simulink model "ServoModel_v5"  (R2021b)
settings: Solver=FixedStepAuto  StartTime=0.0  StopTime=Inf  RelTol=1e-3  EnableMultiTasking=on
libraries: simulink x1, arduinolib x1
settings Model: ExtModeTrigDuration=2  Creator=diego  LastModifiedBy=diego
settings OptimizationCC: EnhancedBackFolding=on  PassReuseOutputArgsAs=Individual arguments  ZeroExternalMemoryAtStartup=off  ZeroInternalMemoryAtStartup=off  MaxStackSize=64  OptimizeBlockOrder=speed  DifferentSizesBufferReuse=on  EfficientTunableParamExpr=on
settings DebuggingCC: ParameterTunabilityLossMsg=error
settings HardwareCC: ProdBitPerInt=16  ProdBitPerPointer=16  ProdBitPerSizeT=16  ProdBitPerPtrDiffT=16  ProdLargestAtomicFloat=None  ProdWordSize=8  ProdHWDeviceType=Atmel->AVR
settings SFSimCC: MATLABDynamicMemAlloc=off
settings RTWCC: Description=Embedded Coder  SystemTargetFile=ert.tlc  HardwareBoard=Arduino Uno  TemplateMakefile=ert_default_tmf  Toolchain=Arduino AVR  BuildConfiguration=Faster Runs
settings CodeAppCC: ForceParamTrailComments=on  IgnoreCustomStorageClasses=off  OperatorAnnotations=on  SimulinkDataObjDesc=on  SFDataObjDesc=on  InsertBlockDesc=on
settings ERTTargetCC: SupportContinuousTime=on  SupportVariableSizeSignals=on  ExtModeTransport=3  ExtModeStaticAlloc=on  ExtModeStaticAllocSize=250  ExtModeMexFile=ext_xcp  ExtModeIntrfLevel=Level2 - Open

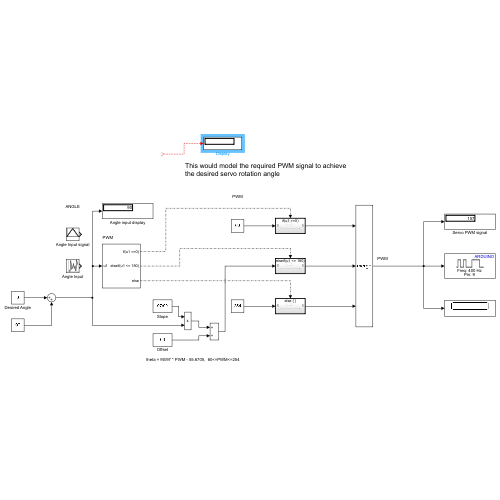
[thumbnail: Simulink's stored preview of the top-level diagram]
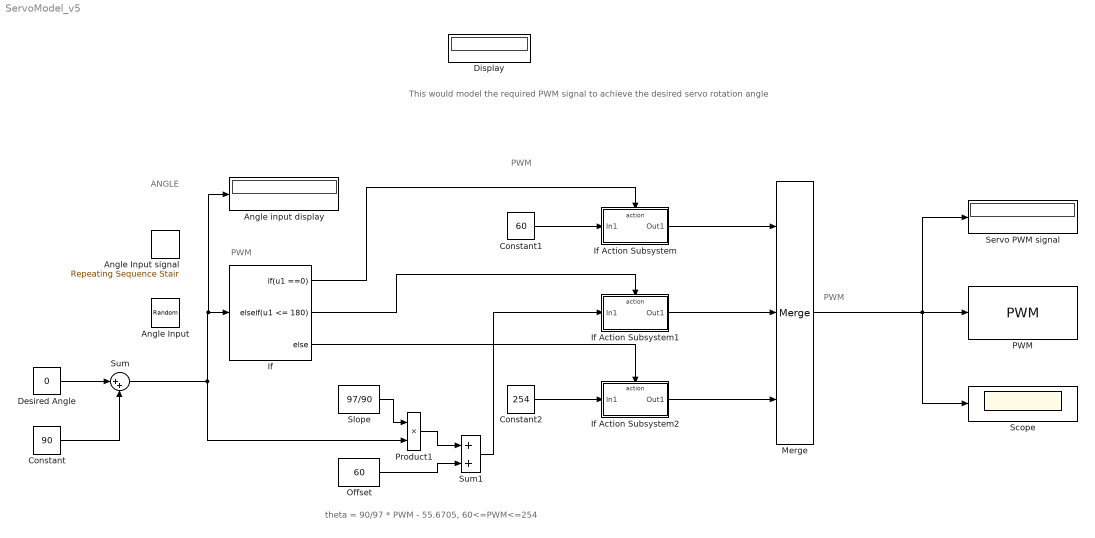
== system ServoModel_v5 ==
  note: This would model the required PWM signal to achieve the desired servo rotation angle
  note: theta = 90/97 * PWM - 55.6705, 60<=PWM<=254
  note: PWM
  note: PWM
  note: PWM
  note: ANGLE
  Angle Input : UniformRandomNumber  Minimum=0  Maximum=180  Seed=66  SampleTime=1.65
  Angle Input signal : simulink/Sources/Repeating Sequence Stair  OutValues=[0:180 179:-1:1]  tsamp=5  OutMin=[0]  OutMax=[255]  OutDataTypeStr=uint8  OutputDataTypeScalingMode=uint8  OutDataType=fixdt(0,8)  ConRadixGroup=Best Precision: Vector-wise  OutScaling=2^-12
  Angle input display : Display
  Constant : Constant  Value=90
  Constant1 : Constant  Value=60
  Constant2 : Constant  Value=254
  Desired Angle : Constant  Value=0
  Display : Display
  If : If  IfExpression=u1 ==0  ElseIfExpressions=u1 <= 180
  If Action Subsystem : Subsystem  TreatAsAtomicUnit=on
  If Action Subsystem1 : Subsystem  TreatAsAtomicUnit=on
  If Action Subsystem2 : Subsystem  TreatAsAtomicUnit=on
  Merge : Merge  Inputs=3
  Offset : Constant  Value=60
  PWM : arduinolib/PWM  pinNumber=9  frequencyType=Specify  desiredFrequency=400  achievableFrequency=400
  Product1 : Product
  Scope : Scope
  Servo PWM signal : Display
  Slope : Constant  Value=97/90
  Sum : Sum  Inputs=|++
  Sum1 : Sum
  wires:
  Offset/1 -> Sum1/2
  Product1/1 -> Sum1/1
  Slope/1 -> Product1/1
  If/1 -> If Action Subsystem/Action
  If/2 -> If Action Subsystem1/Action
  If/3 -> If Action Subsystem2/Action
  If Action Subsystem1/1(Out1) -> Merge/2
  If Action Subsystem/1(Out1) -> Merge/1
  If Action Subsystem2/1(Out1) -> Merge/3
  Merge/1 -> PWM/1, Scope/1, Servo PWM signal/1
  Constant1/1 -> If Action Subsystem/1(In1)
  Constant2/1 -> If Action Subsystem2/1(In1)
  Sum1/1 -> If Action Subsystem1/1(In1)
  Sum/1 -> Product1/2, Angle input display/1, If/1
  Constant/1 -> Sum/2
  Desired Angle/1 -> Sum/1
  ? -> Display/1

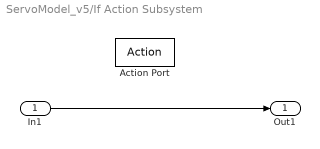
== system ServoModel_v5/If Action Subsystem ==
  In1 : Inport
  Action Port : ActionPort  ActionPortLabel=if(u1 ==0)
  Out1 : Outport
  wires:
  In1/1 -> Out1/1

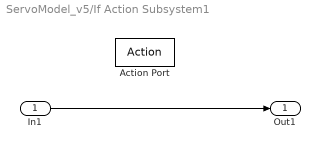
== system ServoModel_v5/If Action Subsystem1 ==
  In1 : Inport
  Action Port : ActionPort  ActionPortLabel=elseif(u1 <= 180)
  Out1 : Outport
  wires:
  In1/1 -> Out1/1

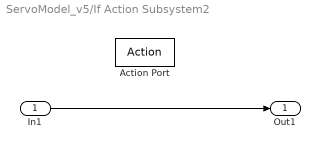
== system ServoModel_v5/If Action Subsystem2 ==
  In1 : Inport
  Action Port : ActionPort  ActionPortLabel=else
  Out1 : Outport
  wires:
  In1/1 -> Out1/1
